simulink model "calcul_SA_SR"  (R2024b)
settings: Solver=FixedStepAuto  StartTime=0.0  StopTime=10.0  FixedStep=Ts  RelTol=1e-3
undefined symbols (not defined in the file or in its folder): epsilon, lf, lr, Re
settings Model: Creator=marti  LastModifiedBy=marti

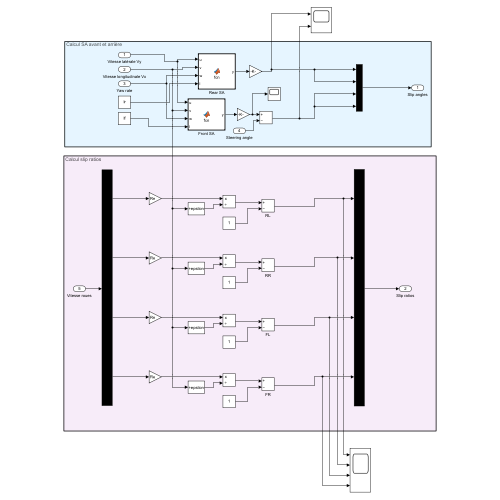
[thumbnail: Simulink's stored preview of the top-level diagram]
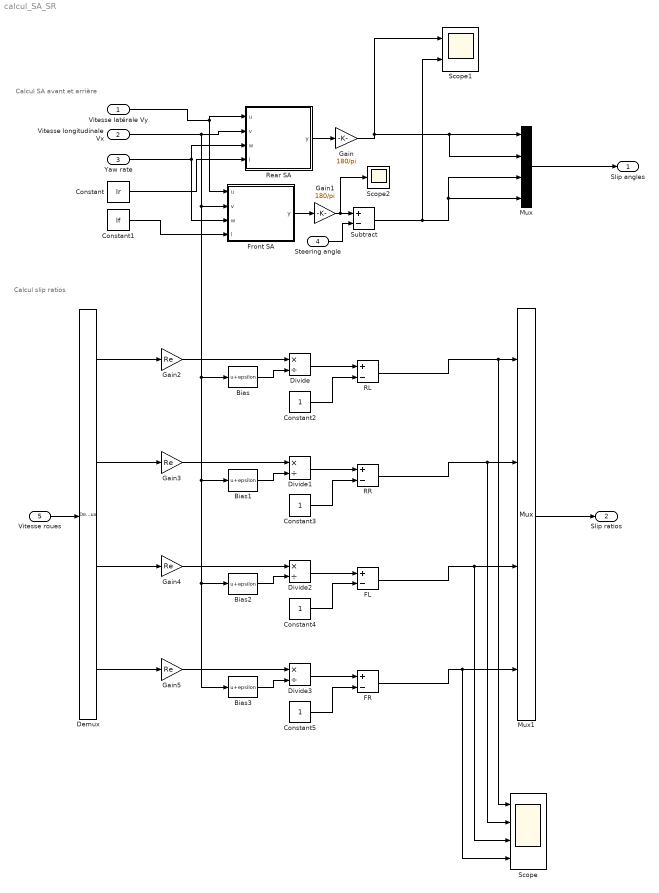
== system calcul_SA_SR ==
  note: Calcul SA avant et arrière
  note: Calcul slip ratios
  Vitesse latérale Vy : Inport
  Vitesse longitudinale Vx : Inport  Port=2
  Yaw rate : Inport  Port=3
  Steering angle : Inport  Port=4
  Vitesse roues : Inport  Port=5
  Bias{,1..3} (4 alike) : Bias  Bias=epsilon  SaturateOnIntegerOverflow=off
  Constant : Constant  Value=lr
  Constant1 : Constant  Value=lf
  Constant{2..5} (4 alike) : Constant
  Demux : Demux
  Divide{,1..3} (4 alike) : Product  Inputs=*/
  FL : Sum  Inputs=+-
  FR : Sum  Inputs=+-
  Front SA : MATLAB Function  TreatAsAtomicUnit=on
  Gain : Gain  Gain=180/pi
  Gain1 : Gain  Gain=180/pi
  Gain{2..5} (4 alike) : Gain  Gain=Re
  Mux : Mux
  Mux1 : Mux
  RL : Sum  Inputs=+-
  RR : Sum  Inputs=+-
  Rear SA : MATLAB Function  TreatAsAtomicUnit=on
  Scope : Scope  NumInputPorts=4
  Scope1 : Scope  NumInputPorts=2
  Scope2 : Scope
  Subtract : Sum  Inputs=+-
  Slip angles : Outport
  Slip ratios : Outport  Port=2
  wires:
  Vitesse latérale Vy/1 -> Front SA/1(u), Rear SA/1(u)
  Rear SA/1(y) -> Gain/1
  Mux/1 -> Slip angles/1
  Mux1/1 -> Slip ratios/1
  Vitesse roues/1 -> Demux/1
  Gain/1 -> Mux/2, Mux/1, Scope1/1
  Yaw rate/1 -> Rear SA/3(w), Front SA/3(w)
  Front SA/1(y) -> Gain1/1
  Gain1/1 -> Scope2/1, Subtract/1
  Steering angle/1 -> Subtract/2
  Subtract/1 -> Scope1/2, Mux/4, Mux/3
  Constant/1 -> Rear SA/4(l)
  Constant1/1 -> Front SA/4(l)
  RL/1 -> Scope/1, Mux1/1
  Divide/1 -> RL/1
  Constant2/1 -> RL/2
  Demux/1 -> Gain2/1
  Gain2/1 -> Divide/1
  Gain3/1 -> Divide1/1
  Divide1/1 -> RR/1
  Constant3/1 -> RR/2
  RR/1 -> Scope/2, Mux1/2
  Demux/2 -> Gain3/1
  Gain4/1 -> Divide2/1
  Divide2/1 -> FL/1
  Constant4/1 -> FL/2
  FL/1 -> Scope/3, Mux1/3
  Demux/3 -> Gain4/1
  Gain5/1 -> Divide3/1
  Divide3/1 -> FR/1
  Constant5/1 -> FR/2
  FR/1 -> Scope/4, Mux1/4
  Demux/4 -> Gain5/1
  Vitesse longitudinale Vx/1 -> Bias3/1, Bias2/1, Bias1/1, Bias/1, Front SA/2(v), Rear SA/2(v)
  Bias/1 -> Divide/2
  Bias1/1 -> Divide1/2
  Bias2/1 -> Divide2/2
  Bias3/1 -> Divide3/2

== matlab function calcul_SA_SR/Front SA ==
  data: u input; y output; v input; w input; l input
function y = fcn(u, v, w, l)

y = atan((u+l*w)/v);
end

== matlab function calcul_SA_SR/Rear SA ==
  data: u input; y output; v input; w input; l input
function y = fcn(u, v, w, l)

y = atan((u-l*w)/v);
end
